simulink model "PD"  (R2024a)
settings: Solver=ode45  StartTime=0.0  StopTime=7  MaxStep=1e-5  RelTol=1e-3  EnableMultiTasking=on
values from neighbouring files (symbols this model uses):
  G = zpk([-10], [0 -2], [5])    [tp2.m]
  Ts = .09    (= 0.09)    [tp2.m]
undefined symbols (not defined in the file or in its folder): PD
libraries: simulink x1
settings Model: Creator=Usuario  LastModifiedBy=Clifferto
settings SolverCC: AlgebraicLoopSolver=TrustRegion
settings DataIOCC: SaveFormat=Array  SignalLoggingSaveFormat=ModelDataLogs  ReturnWorkspaceOutputs=off
settings OptimizationCC: InitFltsAndDblsToZero=on  LifeSpan=inf
settings DebuggingCC: SaveWithParameterizedLinksMsg=none  UnderspecifiedInitializationDetection=Classic  MergeDetectMultiDrivingBlocksExec=none  SignalResolutionControl=TryResolveAllWithWarning  SolverPrmCheckMsg=warning  MultiTaskDSMMsg=warning  MultiTaskCondExecSysMsg=none  FcnCallInpInsideContextMsg=warning  UnconnectedInputMsg=warning  UnconnectedOutputMsg=warning  UnconnectedLineMsg=warning  SFUnexpectedBacktrackingDiag=warning  SFNoUnconditionalDefaultTransitionDiag=warning  SFExecutionAtInitializationDiag=none  ArithmeticOperatorsInVariantConditions=warning
settings HardwareCC: ProdBitPerPointer=32  ProdBitPerSizeT=32  ProdBitPerPtrDiffT=32  ProdLargestAtomicFloat=None  ProdIntDivRoundTo=Undefined  ProdEndianess=Unspecified  ProdWordSize=32  ProdHWDeviceType=32-bit Generic
settings ModelReferenceCC: PropagateSignalLabelsOutOfModel=off
settings SFSimCC: SimUseLocalCustomCode=off  CustomCodeUndefinedFunction=UseInterfaceOnly
settings RTWCC: RTWUseLocalCustomCode=off  GPUComputeCapability=3.5
settings CodeAppCC: StateflowObjectComments=on
settings GRTTargetCC: TargetFcnLib=ansi_tfl_tmw.mat  TargetLangStandard=C89/C90 (ANSI)  CombineOutputUpdateFcns=off  GRTInterface=on
settings ConfigComp: CovMetricSettings=dw  CovSaveCumulativeToWorkspaceVar=on  CovSaveSingleToWorkspaceVar=on  CovExternalEMLEnable=off  CovSFcnEnable=off

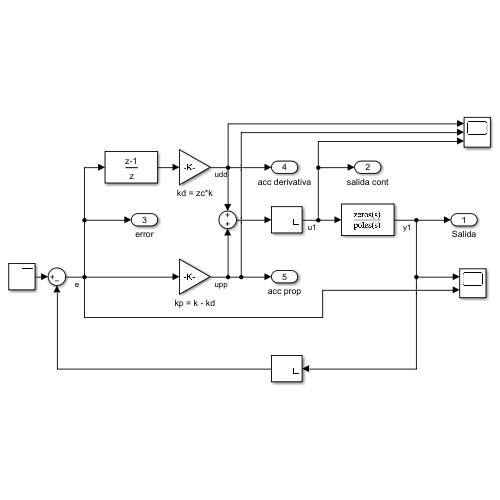
[thumbnail: Simulink's stored preview of the top-level diagram]
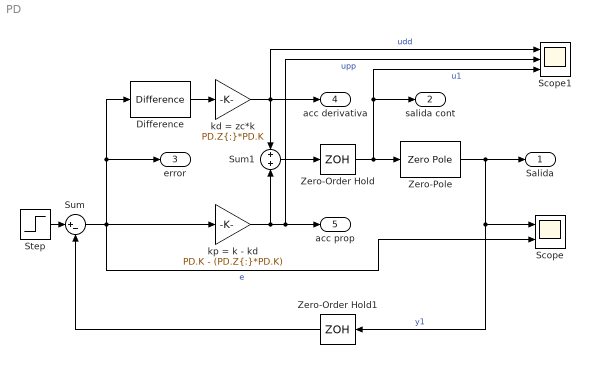
== system PD ==
  Difference : simulink/Discrete/Difference  ICPrevInput=0.0  OutMin=[]  OutMax=[]  OutDataType=fixdt(1, 16)  OutScaling=2^-10  DoSatur=off
  Scope : Scope  NumInputPorts=2
  Scope1 : Scope  NumInputPorts=3
  Step : Step  Time=0  SampleTime=Ts
  Sum : Sum  Inputs=|+-
  Sum1 : Sum
  Zero-Order Hold : ZeroOrderHold  SampleTime=Ts
  Zero-Order Hold1 : ZeroOrderHold  SampleTime=Ts
  Zero-Pole : ZeroPole  Zeros=G.Z{:}  Poles=G.P{:}  Gain=G.K
  kd = zc*k : Gain  Gain=PD.Z{:}*PD.K
  kp = k - kd : Gain  Gain=PD.K - (PD.Z{:}*PD.K)
  Salida : Outport
  salida cont : Outport  Port=2
  error : Outport  Port=3
  acc derivativa : Outport  Port=4
  acc prop : Outport  Port=5
  wires:
  Zero-Order Hold/1 -> Zero-Pole/1, Scope1/3, salida cont/1  "u1"
  Step/1 -> Sum/1
  Zero-Pole/1 -> Zero-Order Hold1/1, Scope/1, Salida/1  "y1"
  kp = k - kd/1 -> Sum1/2, Scope1/2, acc prop/1  "upp"
  Zero-Order Hold1/1 -> Sum/2
  Sum/1 -> kp = k - kd/1, Scope/2, Difference/1, error/1  "e"
  Sum1/1 -> Zero-Order Hold/1
  kd = zc*k/1 -> Scope1/1, acc derivativa/1, Sum1/1  "udd"
  Difference/1 -> kd = zc*k/1
